simulink model "Secondorder"  (Simulink 7.3)
settings: Solver=ode45  StartTime=0.0  StopTime=10.0  RelTol=1e-3
libraries: powerlib x1
settings Model: Creator=srija  LastModifiedBy=srija

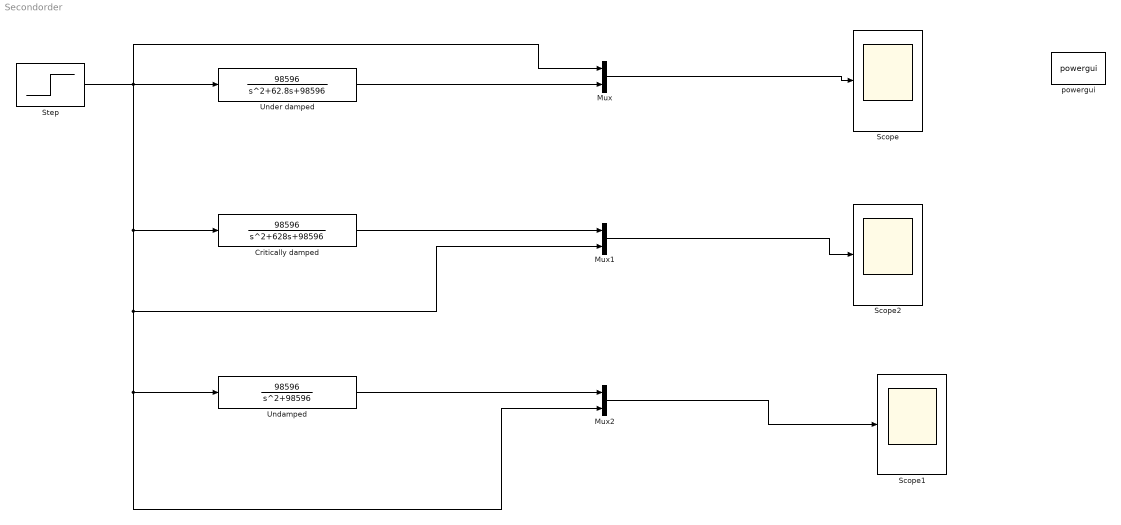
== system Secondorder ==
  Critically damped : TransferFcn  Numerator=[98596]  Denominator=[1 628 98596]
  Mux : Mux  Inputs=2
  Mux1 : Mux  Inputs=2
  Mux2 : Mux  Inputs=2
  Scope : Scope
  Scope1 : Scope
  Scope2 : Scope
      settings: SaveName=ScopeData2
  Step : Step  SampleTime=0
  Undamped : TransferFcn  Numerator=[98596]  Denominator=[1 0 98596]
  Under damped : TransferFcn  Numerator=[98596]  Denominator=[1 62.8 98596]
  powergui : powerlib/powergui  Priority=1  SystemSampleTime=-1  SimulationMode=Continuous  SampleTime=50e-6  frequency=60  SPID=off  DisableSnubberDevices=off  DisableRonSwitches=off  DisableVfSwitches=off  SwTol=0  Interpol=off  frequencyindice=60  echomessages=off  HookPort=off  DisplayEquations=off  FunctionMessages=off  EnableUseOfTLC=off  x0status=blocks  RestoreLinks=warning  Frange=[0:2:500]  Ylog=off  Xlog=on  ShowGrid=off  save=off  variable=ZData  ZoomFFT=on  StartTime=0.0  cycles=1  DisplayStyle=1  fundamental=60  FreqAxis=off  MaxFrequency=1000  frequencyindicesteady=1  RmsSteady=1  display=off  Ts=0  methode=off
  wires:
  Step/1 -> Under damped/1, Mux/1, Critically damped/1, Mux1/2, Undamped/1, Mux2/2
  Under damped/1 -> Mux/2
  Critically damped/1 -> Mux1/1
  Undamped/1 -> Mux2/1
  Mux/1 -> Scope/1
  Mux1/1 -> Scope2/1
  Mux2/1 -> Scope1/1
